simulink model "Uby_lmi"  (R2025b)
settings: Solver=VariableStepAuto  StartTime=0.0  StopTime=10.0  RelTol=1e-3
undefined symbols (not defined in the file): A, B, C, Comp, D, h0, href, K_lmi
settings Model: Creator=Miche  LastModifiedBy=Miche

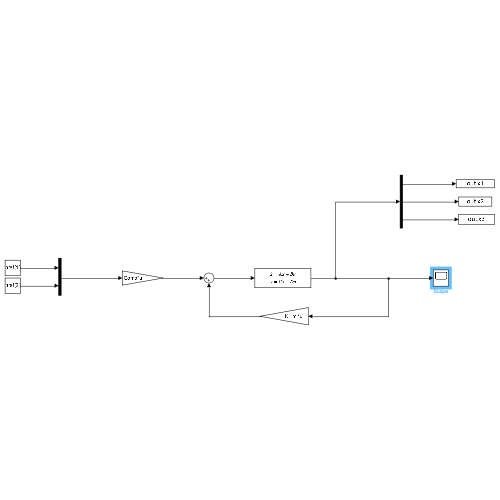
[thumbnail: Simulink's stored preview of the top-level diagram]
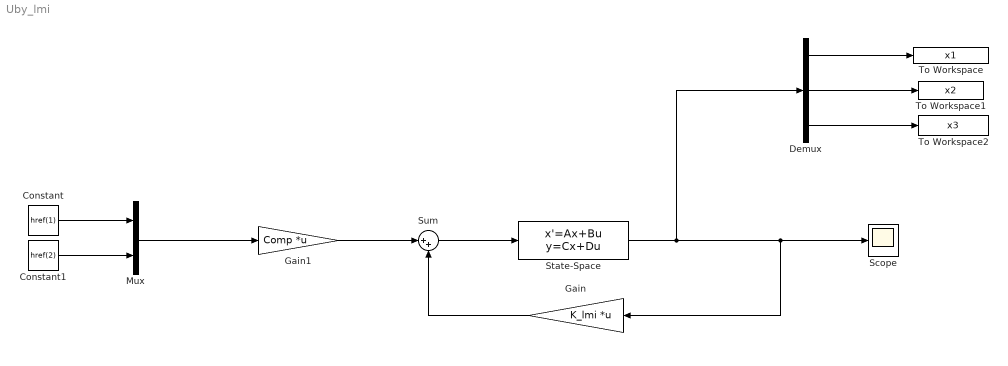
== system Uby_lmi ==
  Constant : Constant  Value=href(1)
  Constant1 : Constant  Value=href(2)
  Demux : Demux  Outputs=3
  Gain : Gain  Gain=K_lmi  Multiplication=Matrix(K*u)
  Gain1 : Gain  Gain=Comp  Multiplication=Matrix(K*u)
  Mux : Mux  Inputs=2
  Scope : Scope
      settings: ActiveDisplayYMinimum=0.048130530012183134  ActiveDisplayYMaximum=0.566825229890352
  State-Space : StateSpace  A=A  B=B  C=C  D=D  InitialCondition=h0
  Sum : Sum  Inputs=|++
  To Workspace : ToWorkspace  VariableName=x1  SaveFormat=Timeseries  SampleTime=-1
  To Workspace1 : ToWorkspace  VariableName=x2  SaveFormat=Timeseries  SampleTime=-1
  To Workspace2 : ToWorkspace  VariableName=x3  SaveFormat=Timeseries  SampleTime=-1
  wires:
  Sum/1 -> State-Space/1
  Gain/1 -> Sum/2
  State-Space/1 -> Demux/1, Gain/1, Scope/1
  Demux/1 -> To Workspace/1
  Demux/2 -> To Workspace1/1
  Demux/3 -> To Workspace2/1
  Gain1/1 -> Sum/1
  Mux/1 -> Gain1/1
  Constant/1 -> Mux/1
  Constant1/1 -> Mux/2
